simulink model "pi_controller"  (R2022a)
settings: Solver=VariableStepAuto  StartTime=0.0  StopTime=10.0  RelTol=1e-3
settings Model: Creator=Laptop-Academy.com  LastModifiedBy=Laptop-Academy.com

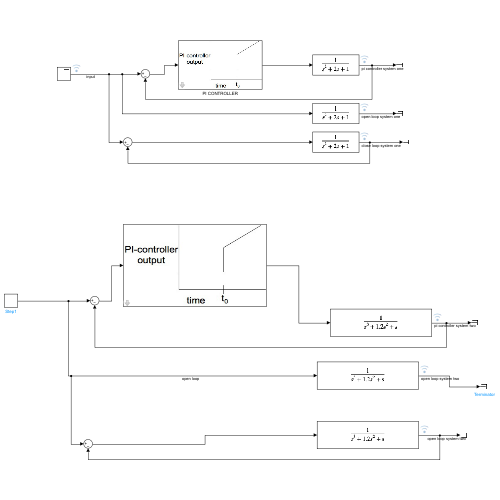
[thumbnail: Simulink's stored preview of the top-level diagram]
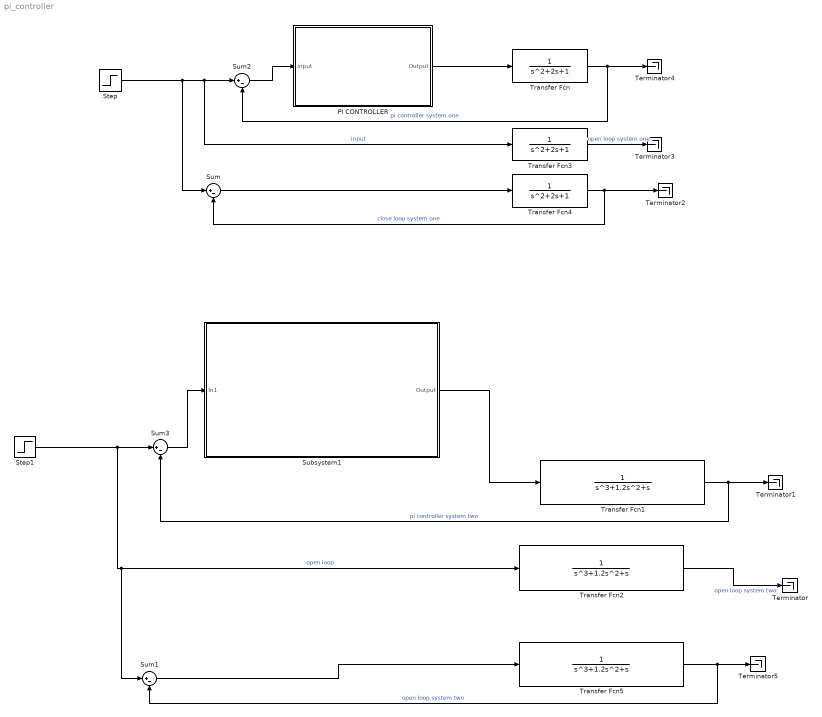
== system pi_controller ==
  PI CONTROLLER : Subsystem  mask{p=1, i=0.1}
      mask prompts: p "probortianal gain (p)"; i "integral gain (i)"
      mask Display: image("F:\os_academy_labs\pid_controller\media\pi.jpg");
  Step : Step  SampleTime=0
  Step1 : Step  SampleTime=0
  Subsystem1 : Subsystem  mask{p=5, i=0.5}
      mask prompts: p "probortional gain (p)"; i "integral gain (i)"
      mask Display: image("F:\os_academy_labs\pid_controller\media\pi.jpg");
  Sum{,1..3} (4 alike) : Sum  Inputs=|+-
  Terminator{,1..5} (6 alike) : Terminator
  Transfer Fcn : TransferFcn
  Transfer Fcn1 : TransferFcn  Denominator=[1 1.2 1 0]
  Transfer Fcn2 : TransferFcn  Denominator=[1 1.2 1 0]
  Transfer Fcn3 : TransferFcn
  Transfer Fcn4 : TransferFcn
  Transfer Fcn5 : TransferFcn  Denominator=[1 1.2 1 0]
  wires:
  Step/1 -> Sum/1, Sum2/1, Transfer Fcn3/1  "input"
  Step1/1 -> Sum1/1, Transfer Fcn2/1, Sum3/1  "open loop"
  PI CONTROLLER/1(Output) -> Transfer Fcn/1
  Subsystem1/1(Output) -> Transfer Fcn1/1
  Transfer Fcn2/1 -> Terminator/1  "open loop system two"
  Transfer Fcn1/1 -> Sum3/2, Terminator1/1  "pi controller system two"
  Sum/1 -> Transfer Fcn4/1
  Transfer Fcn4/1 -> Terminator2/1, Sum/2  "close loop system one"
  Transfer Fcn3/1 -> Terminator3/1  "open loop system one"
  Transfer Fcn/1 -> Sum2/2, Terminator4/1  "pi controller system one"
  Sum1/1 -> Transfer Fcn5/1
  Transfer Fcn5/1 -> Terminator5/1, Sum1/2  "open loop system two"
  Sum2/1 -> PI CONTROLLER/1(input)
  Sum3/1 -> Subsystem1/1(In1)

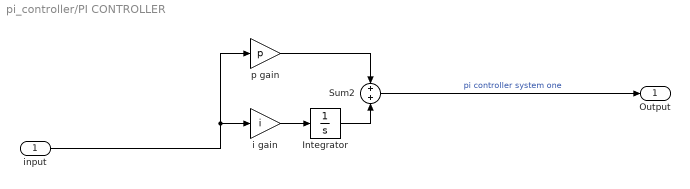
== system pi_controller/PI CONTROLLER ==
  input : Inport
  Integrator : Integrator
  Sum2 : Sum  Inputs=+|+
  i gain : Gain  Gain=i
  p gain : Gain  Gain=p
  Output : Outport
  wires:
  input/1 -> p gain/1, i gain/1
  Sum2/1 -> Output/1  "pi controller system one"
  i gain/1 -> Integrator/1
  Integrator/1 -> Sum2/2
  p gain/1 -> Sum2/1

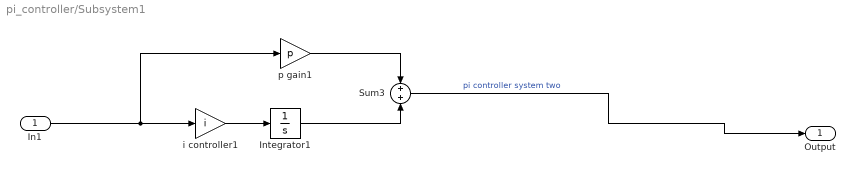
== system pi_controller/Subsystem1 ==
  In1 : Inport
  Integrator1 : Integrator
  Sum3 : Sum  Inputs=+|+
  i controller1 : Gain  Gain=i
  p gain1 : Gain  Gain=p
  Output : Outport
  wires:
  Integrator1/1 -> Sum3/2
  In1/1 -> p gain1/1, i controller1/1
  Sum3/1 -> Output/1  "pi controller system two"
  i controller1/1 -> Integrator1/1
  p gain1/1 -> Sum3/1
